simulink model "gm_flyback_dt_vnl"  (R2021b)
settings: Solver=FixedStepDiscrete  StartTime=0.0  StopTime=100e-3  RelTol=1e-3
undefined symbols (not defined in the file or in its folder): DiscIntNeverNeededParam
libraries: simulink x5
Description:
  | Symmetric FIR Filter
  | This example shows how to use HDL Coder(TM) to check, generate,
  | and verify HDL for a fixed-point symmetric FIR filter.
settings Model: Creator=The MathWorks, Inc.  LastModifiedBy=Marco Milanesi
settings SolverCC: AlgebraicLoopSolver=TrustRegion  AutoInsertRateTranBlk=on
settings DataIOCC: LimitDataPoints=on  SaveFormat=Array  SaveOutput=off  SignalLogging=off  SaveTime=off  ReturnWorkspaceOutputs=off  SignalLoggingName=logsOut
settings OptimizationCC: BlockReduction=off  BooleanDataType=off  ConditionallyExecuteInputs=off  DefaultParameterBehavior=Inlined  InheritOutputTypeSmallerThanSingle=on  InlineInvariantSignals=on  ExpressionDepthLimit=2147483647  InitFltsAndDblsToZero=on  LifeSpan=inf  BufferReusableBoundary=off
settings DebuggingCC: AlgebraicLoopMsg=error  SaveWithParameterizedLinksMsg=none  UnderspecifiedInitializationDetection=Classic  MergeDetectMultiDrivingBlocksExec=none  CheckExecutionContextPreStartOutputMsg=on  SignalResolutionControl=TryResolveAllWithWarning  InheritedTsInSrcMsg=none  MultiTaskDSMMsg=warning  MultiTaskCondExecSysMsg=none  SingleTaskRateTransMsg=error  IntegerOverflowMsg=none  ParameterPrecisionLossMsg=none  FcnCallInpInsideContextMsg=warning  BusObjectLabelMismatch=none  StateNameClashWarn=warning  SFUnexpectedBacktrackingDiag=warning  SFNoUnconditionalDefaultTransitionDiag=warning  SFExecutionAtInitializationDiag=none  SFMachineParentedDataDiag=warning  IntegerSaturationMsg=none  ArithmeticOperatorsInVariantConditions=warning
settings HardwareCC: ProdBitPerPointer=32  ProdBitPerSizeT=32  ProdBitPerPtrDiffT=32  ProdLargestAtomicFloat=None  ProdIntDivRoundTo=Undefined  ProdEndianess=Unspecified  ProdWordSize=32  ProdHWDeviceType=ASIC/FPGA  TargetUnknown=on  ProdEqTarget=off
settings ModelReferenceCC: PropagateSignalLabelsOutOfModel=off
settings SFSimCC: SimUseLocalCustomCode=off  CustomCodeUndefinedFunction=UseInterfaceOnly
settings RTWCC: RTWUseLocalCustomCode=off
settings CodeAppCC: StateflowObjectComments=on
settings GRTTargetCC: TargetFcnLib=ansi_tfl_tmw.mat  TargetLangStandard=C89/C90 (ANSI)  CombineOutputUpdateFcns=off  GRTInterface=on
settings ConfigComp: CovMetricSettings=dw  CovSaveCumulativeToWorkspaceVar=on  CovSaveSingleToWorkspaceVar=on  CovExternalEMLEnable=off

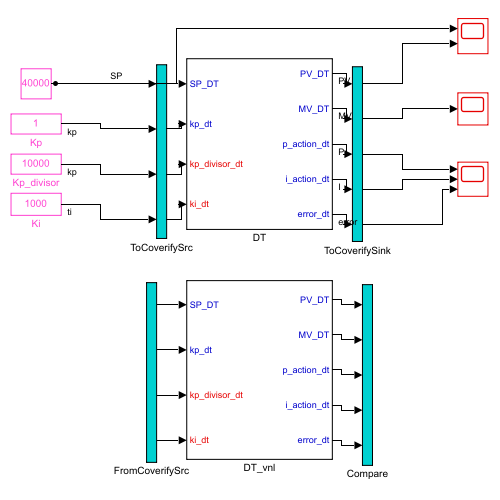
[thumbnail: Simulink's stored preview of the top-level diagram]
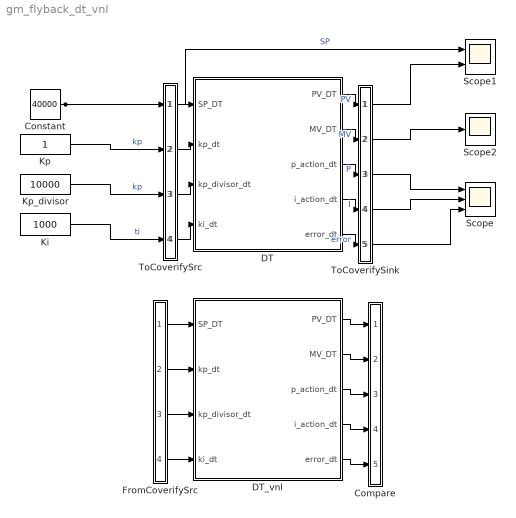
== system gm_flyback_dt_vnl ==
  Compare : Subsystem
      mask Display: disp('')
  Constant : Constant  Value=40000  OutDataTypeStr=fixdt(1,64,32)
  DT : Subsystem
  DT_vnl : Subsystem
  FromCoverifySrc : Subsystem
      mask Display: disp('')
  Ki : Constant  Value=1000  OutDataTypeStr=fixdt(1,64,32)
  Kp : Constant  OutDataTypeStr=fixdt(1,64,32)
  Kp_divisor : Constant  Value=10000  OutDataTypeStr=fixdt(1,64,32)
  Scope : Scope  NumInputPorts=3
  Scope1 : Scope  NumInputPorts=2
  Scope2 : Scope
  ToCoverifySink : Subsystem
      mask Display: disp('')
  ToCoverifySrc : Subsystem
      mask Display: disp('')
  wires:
  Constant/1 -> Scope1/1, ToCoverifySrc/1(in1)  "SP"
  ToCoverifySrc/1(out1) -> DT/1(SP_DT)
  ToCoverifySrc/2(out2) -> DT/2(kp_dt)
  ToCoverifySrc/3(out3) -> DT/3(kp_divisor_dt)
  ToCoverifySrc/4(out4) -> DT/4(ki_dt)
  DT/1(PV_DT) -> ToCoverifySink/1(in1)  "PV"
  DT/2(MV_DT) -> ToCoverifySink/2(in2)  "MV"
  DT/3(p_action_dt) -> ToCoverifySink/3(in3)  "P"
  DT/4(i_action_dt) -> ToCoverifySink/4(in4)  "I"
  DT/5(error_dt) -> ToCoverifySink/5(in5)  "error"
  Kp/1 -> ToCoverifySrc/2(in2)  "kp"
  Kp_divisor/1 -> ToCoverifySrc/3(in3)  "kp"
  Ki/1 -> ToCoverifySrc/4(in4)  "ti"
  ToCoverifySink/1(out1) -> Scope1/2
  ToCoverifySink/2(out2) -> Scope2/1
  ToCoverifySink/3(out3) -> Scope/1
  ToCoverifySink/4(out4) -> Scope/2
  ToCoverifySink/5(out5) -> Scope/3
  FromCoverifySrc/1(out1) -> DT_vnl/1(SP_DT)
  FromCoverifySrc/2(out2) -> DT_vnl/2(kp_dt)
  FromCoverifySrc/3(out3) -> DT_vnl/3(kp_divisor_dt)
  FromCoverifySrc/4(out4) -> DT_vnl/4(ki_dt)
  DT_vnl/1(PV_DT) -> Compare/1(in1)
  DT_vnl/2(MV_DT) -> Compare/2(in2)
  DT_vnl/3(p_action_dt) -> Compare/3(in3)
  DT_vnl/4(i_action_dt) -> Compare/4(in4)
  DT_vnl/5(error_dt) -> Compare/5(in5)

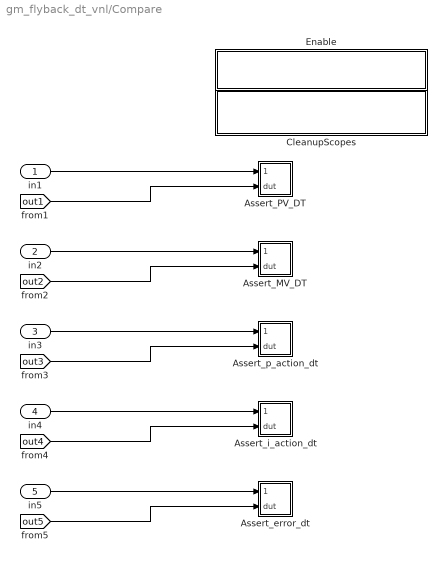
== system gm_flyback_dt_vnl/Compare ==
  in1 : Inport
  in2 : Inport  Port=2
  in3 : Inport  Port=3
  in4 : Inport  Port=4
  in5 : Inport  Port=5
  Assert_MV_DT : Subsystem
  Assert_PV_DT : Subsystem
  Assert_error_dt : Subsystem
  Assert_i_action_dt : Subsystem
  Assert_p_action_dt : Subsystem
  CleanupScopes : Subsystem
      settings: OpenFcn=|
      | blkName = gcb; %self block
      | idx = regexp(blkName, '/CleanupScopes$', 'once');
      | blkParent = blkName(1:idx-1);
      | blks=find_system(blkParent, 'LookUnderMasks', 'all','blocktype', 'Scope');
      | for itr = 1:length(blks)
      | 	 hScopeCfg = get_param(blks{itr},'ScopeConfiguration');
      | 	 hScopeCfg.Visible = ~ hScopeCfg.Visible;
      | end
      | drawnow;
      mask Display: fprintf(message('hdlcoder:cosim:vnl_dblclick').getString());
  Enable : Subsystem
      settings: OpenFcn=|
      | blkName = gcb;
      | idx = regexp(blkName, '/Enable$', 'once');
      | blkParent = blkName(1:idx-1);
      | blks=find_system(blkParent, 'LookUnderMasks', 'all','blocktype', 'Assertion');
      | e = get_param(blks{1}, 'Enabled');
      | if strcmp(e, 'on'), f= 'off';, else, f = 'on';, end
      | for ii=1:length(blks), set_param(blks{ii}, 'Enabled', f);, end
      | set_param(gcb, 'MaskDisplay',['fprintf(message(''hdlcoder:cosim:vnl_dblclick_assertions'',','''',upper(e),'''',').getString())']);
      mask Display: fprintf(message('hdlcoder:cosim:vnl_dblclick_assertions','OFF').getString());
  wires:
  in1/1 -> Assert_PV_DT/1(cosim)
  [out1] -> Assert_PV_DT/2(dut)
  in2/1 -> Assert_MV_DT/1(cosim)
  [out2] -> Assert_MV_DT/2(dut)
  in3/1 -> Assert_p_action_dt/1(cosim)
  [out3] -> Assert_p_action_dt/2(dut)
  in4/1 -> Assert_i_action_dt/1(cosim)
  [out4] -> Assert_i_action_dt/2(dut)
  in5/1 -> Assert_error_dt/1(cosim)
  [out5] -> Assert_error_dt/2(dut)

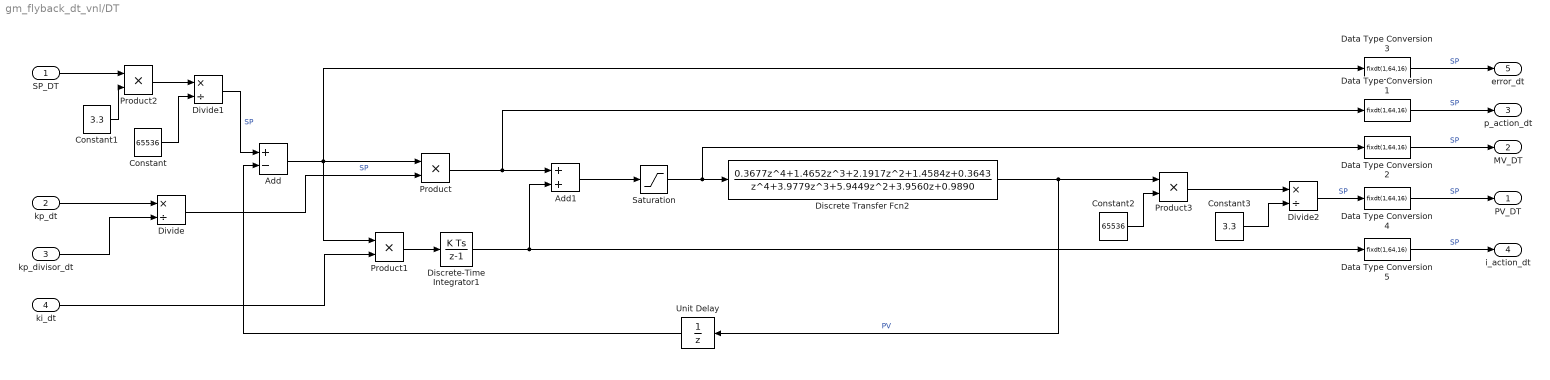
== system gm_flyback_dt_vnl/DT ==
  SP_DT : Inport  OutDataTypeStr=fixdt(1,64,32)  SampleTime=0.00001
  kp_dt : Inport  Port=2  OutDataTypeStr=fixdt(1,64,32)  SampleTime=0.00001
  kp_divisor_dt : Inport  Port=3  OutDataTypeStr=fixdt(1,64,32)  SampleTime=0.00001
  ki_dt : Inport  Port=4  OutDataTypeStr=fixdt(1,64,32)  SampleTime=0.00001
  Add : Sum  Inputs=+-  AccumDataTypeStr=fixdt(1,64,32)  OutDataTypeStr=fixdt(1,64,32)
  Add1 : Sum  AccumDataTypeStr=fixdt(1,64,32)  OutDataTypeStr=fixdt(1,64,32)
  Constant : Constant  Value=65536  OutDataTypeStr=fixdt(1,64,32)
  Constant1 : Constant  Value=3.3  OutDataTypeStr=fixdt(1,64,32)
  Constant2 : Constant  Value=65536  OutDataTypeStr=fixdt(1,64,32)
  Constant3 : Constant  Value=3.3  OutDataTypeStr=fixdt(1,64,32)
  Data Type Conversion{1..5} (5 alike) : DataTypeConversion  OutDataTypeStr=fixdt(1,64,16)
  Discrete Transfer Fcn2 : DiscreteTransferFcn  Numerator=[0.3677 1.4652 2.1917 1.4584 0.3643]  Denominator=[1 3.9779 5.9449 3.9560 0.9890]  SampleTime=0.00001  NumCoefDataTypeStr=fixdt(1,64,32)  DenCoefDataTypeStr=fixdt(1,64,32)  NumProductDataTypeStr=fixdt(1,64,32)  DenProductDataTypeStr=fixdt(1,64,32)  NumAccumDataTypeStr=fixdt(1,64,32)  DenAccumDataTypeStr=fixdt(1,64,32)  OutDataTypeStr=fixdt(1,64,32)
  Discrete-Time Integrator1 : DiscreteIntegrator  SampleTime=0.00001  OutDataTypeStr=fixdt(1,64,32)  ICPrevOutput=DiscIntNeverNeededParam  ICPrevScaledInput=DiscIntNeverNeededParam
  Divide : Product  Inputs=*/  RndMeth=Zero  SaturateOnIntegerOverflow=on  LockScale=on
  Divide1 : Product  Inputs=*/  RndMeth=Zero  SaturateOnIntegerOverflow=on  LockScale=on
  Divide2 : Product  Inputs=*/  RndMeth=Zero  SaturateOnIntegerOverflow=on  LockScale=on
  Product{,1..3} (4 alike) : Product  OutDataTypeStr=fixdt(1,64,32)
  Saturation : Saturate  UpperLimit=255  LowerLimit=0  OutDataTypeStr=fixdt(1,64,32)
  Unit Delay : UnitDelay  SampleTime=0.00001  HasFrameUpgradeWarning=on
  PV_DT : Outport  OutDataTypeStr=fixdt(1,64,16)  SampleTime=0.00001  VectorParamsAs1DForOutWhenUnconnected=off
  MV_DT : Outport  Port=2  OutDataTypeStr=fixdt(1,64,16)  SampleTime=0.00001  VectorParamsAs1DForOutWhenUnconnected=off
  p_action_dt : Outport  Port=3  OutDataTypeStr=fixdt(1,64,16)  SampleTime=0.00001  VectorParamsAs1DForOutWhenUnconnected=off
  i_action_dt : Outport  Port=4  OutDataTypeStr=fixdt(1,64,16)  SampleTime=0.00001  VectorParamsAs1DForOutWhenUnconnected=off
  error_dt : Outport  Port=5  OutDataTypeStr=fixdt(1,64,16)  SampleTime=0.00001  VectorParamsAs1DForOutWhenUnconnected=off
  wires:
  Unit Delay/1 -> Add/2
  Product1/1 -> Discrete-Time Integrator1/1
  Add/1 -> Data Type Conversion3/1, Product/1, Product1/1
  Product/1 -> Data Type Conversion1/1, Add1/1
  Discrete Transfer Fcn2/1 -> Product3/1, Unit Delay/1  "PV"
  Discrete-Time Integrator1/1 -> Data Type Conversion5/1, Add1/2
  Data Type Conversion1/1 -> p_action_dt/1  "SP"
  Data Type Conversion3/1 -> error_dt/1  "SP"
  Data Type Conversion2/1 -> MV_DT/1  "SP"
  Data Type Conversion4/1 -> PV_DT/1  "SP"
  Data Type Conversion5/1 -> i_action_dt/1  "SP"
  ki_dt/1 -> Product1/2
  kp_dt/1 -> Divide/1
  kp_divisor_dt/1 -> Divide/2
  Divide/1 -> Product/2  "SP"
  Add1/1 -> Saturation/1
  Saturation/1 -> Discrete Transfer Fcn2/1, Data Type Conversion2/1
  SP_DT/1 -> Product2/1
  Product2/1 -> Divide1/1
  Divide1/1 -> Add/1  "SP"
  Constant/1 -> Divide1/2
  Constant1/1 -> Product2/2
  Product3/1 -> Divide2/1
  Constant2/1 -> Product3/2
  Constant3/1 -> Divide2/2
  Divide2/1 -> Data Type Conversion4/1  "SP"

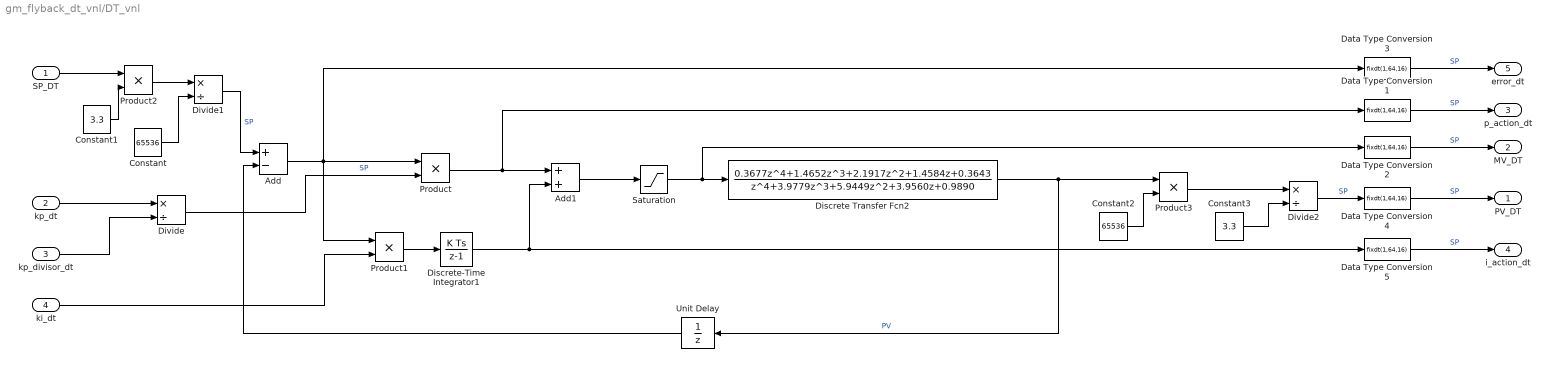
== system gm_flyback_dt_vnl/DT_vnl ==
  SP_DT : Inport  OutDataTypeStr=fixdt(1,64,32)  SampleTime=0.00001
  kp_dt : Inport  Port=2  OutDataTypeStr=fixdt(1,64,32)  SampleTime=0.00001
  kp_divisor_dt : Inport  Port=3  OutDataTypeStr=fixdt(1,64,32)  SampleTime=0.00001
  ki_dt : Inport  Port=4  OutDataTypeStr=fixdt(1,64,32)  SampleTime=0.00001
  Add : Sum  Inputs=+-  AccumDataTypeStr=fixdt(1,64,32)  OutDataTypeStr=fixdt(1,64,32)
  Add1 : Sum  AccumDataTypeStr=fixdt(1,64,32)  OutDataTypeStr=fixdt(1,64,32)
  Constant : Constant  Value=65536  OutDataTypeStr=fixdt(1,64,32)
  Constant1 : Constant  Value=3.3  OutDataTypeStr=fixdt(1,64,32)
  Constant2 : Constant  Value=65536  OutDataTypeStr=fixdt(1,64,32)
  Constant3 : Constant  Value=3.3  OutDataTypeStr=fixdt(1,64,32)
  Data Type Conversion{1..5} (5 alike) : DataTypeConversion  OutDataTypeStr=fixdt(1,64,16)
  Discrete Transfer Fcn2 : DiscreteTransferFcn  Numerator=[0.3677 1.4652 2.1917 1.4584 0.3643]  Denominator=[1 3.9779 5.9449 3.9560 0.9890]  SampleTime=0.00001  NumCoefDataTypeStr=fixdt(1,64,32)  DenCoefDataTypeStr=fixdt(1,64,32)  NumProductDataTypeStr=fixdt(1,64,32)  DenProductDataTypeStr=fixdt(1,64,32)  NumAccumDataTypeStr=fixdt(1,64,32)  DenAccumDataTypeStr=fixdt(1,64,32)  OutDataTypeStr=fixdt(1,64,32)
  Discrete-Time Integrator1 : DiscreteIntegrator  SampleTime=0.00001  OutDataTypeStr=fixdt(1,64,32)  ICPrevOutput=DiscIntNeverNeededParam  ICPrevScaledInput=DiscIntNeverNeededParam
  Divide : Product  Inputs=*/  RndMeth=Zero  SaturateOnIntegerOverflow=on  LockScale=on
  Divide1 : Product  Inputs=*/  RndMeth=Zero  SaturateOnIntegerOverflow=on  LockScale=on
  Divide2 : Product  Inputs=*/  RndMeth=Zero  SaturateOnIntegerOverflow=on  LockScale=on
  Product{,1..3} (4 alike) : Product  OutDataTypeStr=fixdt(1,64,32)
  Saturation : Saturate  UpperLimit=255  LowerLimit=0  OutDataTypeStr=fixdt(1,64,32)
  Unit Delay : UnitDelay  SampleTime=0.00001  HasFrameUpgradeWarning=on
  PV_DT : Outport  OutDataTypeStr=fixdt(1,64,16)  SampleTime=0.00001  VectorParamsAs1DForOutWhenUnconnected=off
  MV_DT : Outport  Port=2  OutDataTypeStr=fixdt(1,64,16)  SampleTime=0.00001  VectorParamsAs1DForOutWhenUnconnected=off
  p_action_dt : Outport  Port=3  OutDataTypeStr=fixdt(1,64,16)  SampleTime=0.00001  VectorParamsAs1DForOutWhenUnconnected=off
  i_action_dt : Outport  Port=4  OutDataTypeStr=fixdt(1,64,16)  SampleTime=0.00001  VectorParamsAs1DForOutWhenUnconnected=off
  error_dt : Outport  Port=5  OutDataTypeStr=fixdt(1,64,16)  SampleTime=0.00001  VectorParamsAs1DForOutWhenUnconnected=off
  wires:
  Divide2/1 -> Data Type Conversion4/1  "SP"
  Constant3/1 -> Divide2/2
  Constant2/1 -> Product3/2
  Product3/1 -> Divide2/1
  Constant1/1 -> Product2/2
  Constant/1 -> Divide1/2
  Divide1/1 -> Add/1  "SP"
  Product2/1 -> Divide1/1
  SP_DT/1 -> Product2/1
  Saturation/1 -> Data Type Conversion2/1, Discrete Transfer Fcn2/1
  Add1/1 -> Saturation/1
  Divide/1 -> Product/2  "SP"
  kp_divisor_dt/1 -> Divide/2
  kp_dt/1 -> Divide/1
  ki_dt/1 -> Product1/2
  Data Type Conversion5/1 -> i_action_dt/1  "SP"
  Data Type Conversion4/1 -> PV_DT/1  "SP"
  Data Type Conversion2/1 -> MV_DT/1  "SP"
  Data Type Conversion3/1 -> error_dt/1  "SP"
  Data Type Conversion1/1 -> p_action_dt/1  "SP"
  Discrete-Time Integrator1/1 -> Add1/2, Data Type Conversion5/1
  Discrete Transfer Fcn2/1 -> Unit Delay/1, Product3/1  "PV"
  Product/1 -> Add1/1, Data Type Conversion1/1
  Add/1 -> Product1/1, Product/1, Data Type Conversion3/1
  Product1/1 -> Discrete-Time Integrator1/1
  Unit Delay/1 -> Add/2

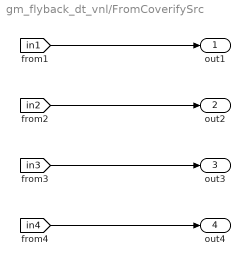
== system gm_flyback_dt_vnl/FromCoverifySrc ==
  out1 : Outport
  out2 : Outport  Port=2
  out3 : Outport  Port=3
  out4 : Outport  Port=4
  wires:
  [in1] -> out1/1
  [in2] -> out2/1
  [in3] -> out3/1
  [in4] -> out4/1

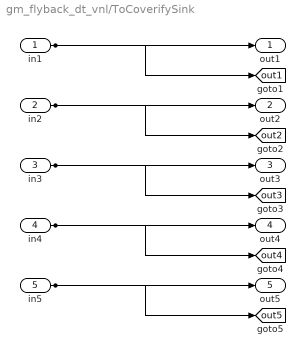
== system gm_flyback_dt_vnl/ToCoverifySink ==
  in1 : Inport
  in2 : Inport  Port=2
  in3 : Inport  Port=3
  in4 : Inport  Port=4
  in5 : Inport  Port=5
  out1 : Outport
  out2 : Outport  Port=2
  out3 : Outport  Port=3
  out4 : Outport  Port=4
  out5 : Outport  Port=5
  tag scope: out1=global, out2=global, out3=global, out4=global, out5=global
  wires:
  in1/1 -> out1/1, [out1]
  in2/1 -> out2/1, [out2]
  in3/1 -> out3/1, [out3]
  in4/1 -> out4/1, [out4]
  in5/1 -> out5/1, [out5]

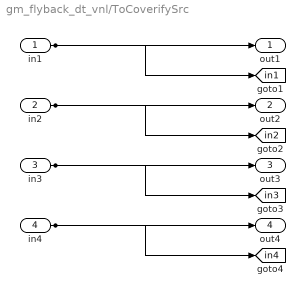
== system gm_flyback_dt_vnl/ToCoverifySrc ==
  in1 : Inport
  in2 : Inport  Port=2
  in3 : Inport  Port=3
  in4 : Inport  Port=4
  out1 : Outport
  out2 : Outport  Port=2
  out3 : Outport  Port=3
  out4 : Outport  Port=4
  tag scope: in1=global, in2=global, in3=global, in4=global
  wires:
  in1/1 -> out1/1, [in1]
  in2/1 -> out2/1, [in2]
  in3/1 -> out3/1, [in3]
  in4/1 -> out4/1, [in4]

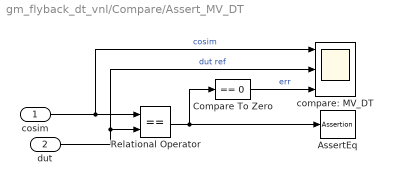
== system gm_flyback_dt_vnl/Compare/Assert_MV_DT ==
  cosim : Inport
  dut : Inport  Port=2
  AssertEq : Assertion  StopWhenAssertionFail=off
  Compare To Zero : simulink/Logic and Bit Operations/Compare To Zero  relop===  OutDataTypeStr=boolean
  Relational Operator : RelationalOperator  Operator===  OutDataTypeStr=boolean  RndMeth=Nearest
  compare: MV_DT : Scope  NumInputPorts=3
  wires:
  Compare To Zero/1 -> compare: MV_DT/3  "err"
  Relational Operator/1 -> Compare To Zero/1, AssertEq/1
  cosim/1 -> compare: MV_DT/1, Relational Operator/1  "cosim"
  dut/1 -> compare: MV_DT/2, Relational Operator/2  "dut ref"

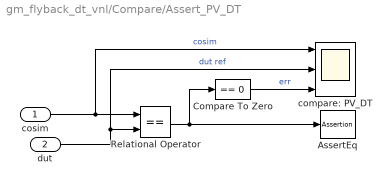
== system gm_flyback_dt_vnl/Compare/Assert_PV_DT ==
  cosim : Inport
  dut : Inport  Port=2
  AssertEq : Assertion  StopWhenAssertionFail=off
  Compare To Zero : simulink/Logic and Bit Operations/Compare To Zero  relop===  OutDataTypeStr=boolean
  Relational Operator : RelationalOperator  Operator===  OutDataTypeStr=boolean  RndMeth=Nearest
  compare: PV_DT : Scope  NumInputPorts=3
  wires:
  Compare To Zero/1 -> compare: PV_DT/3  "err"
  Relational Operator/1 -> Compare To Zero/1, AssertEq/1
  cosim/1 -> compare: PV_DT/1, Relational Operator/1  "cosim"
  dut/1 -> compare: PV_DT/2, Relational Operator/2  "dut ref"

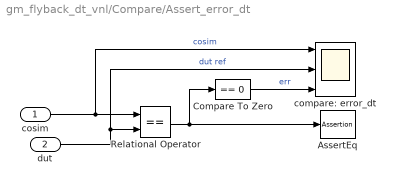
== system gm_flyback_dt_vnl/Compare/Assert_error_dt ==
  cosim : Inport
  dut : Inport  Port=2
  AssertEq : Assertion  StopWhenAssertionFail=off
  Compare To Zero : simulink/Logic and Bit Operations/Compare To Zero  relop===  OutDataTypeStr=boolean
  Relational Operator : RelationalOperator  Operator===  OutDataTypeStr=boolean  RndMeth=Nearest
  compare: error_dt : Scope  NumInputPorts=3
  wires:
  Compare To Zero/1 -> compare: error_dt/3  "err"
  Relational Operator/1 -> Compare To Zero/1, AssertEq/1
  cosim/1 -> compare: error_dt/1, Relational Operator/1  "cosim"
  dut/1 -> compare: error_dt/2, Relational Operator/2  "dut ref"

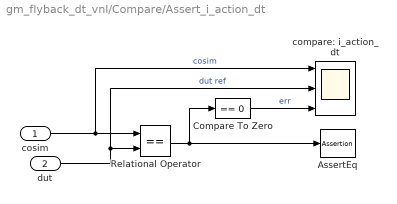
== system gm_flyback_dt_vnl/Compare/Assert_i_action_dt ==
  cosim : Inport
  dut : Inport  Port=2
  AssertEq : Assertion  StopWhenAssertionFail=off
  Compare To Zero : simulink/Logic and Bit Operations/Compare To Zero  relop===  OutDataTypeStr=boolean
  Relational Operator : RelationalOperator  Operator===  OutDataTypeStr=boolean  RndMeth=Nearest
  compare: i_action_dt : Scope  NumInputPorts=3
  wires:
  Compare To Zero/1 -> compare: i_action_dt/3  "err"
  Relational Operator/1 -> Compare To Zero/1, AssertEq/1
  cosim/1 -> compare: i_action_dt/1, Relational Operator/1  "cosim"
  dut/1 -> compare: i_action_dt/2, Relational Operator/2  "dut ref"

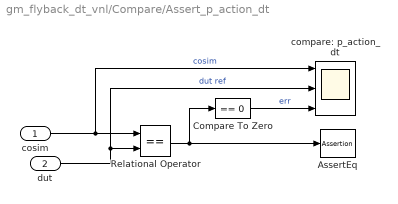
== system gm_flyback_dt_vnl/Compare/Assert_p_action_dt ==
  cosim : Inport
  dut : Inport  Port=2
  AssertEq : Assertion  StopWhenAssertionFail=off
  Compare To Zero : simulink/Logic and Bit Operations/Compare To Zero  relop===  OutDataTypeStr=boolean
  Relational Operator : RelationalOperator  Operator===  OutDataTypeStr=boolean  RndMeth=Nearest
  compare: p_action_dt : Scope  NumInputPorts=3
  wires:
  Compare To Zero/1 -> compare: p_action_dt/3  "err"
  Relational Operator/1 -> Compare To Zero/1, AssertEq/1
  cosim/1 -> compare: p_action_dt/1, Relational Operator/1  "cosim"
  dut/1 -> compare: p_action_dt/2, Relational Operator/2  "dut ref"

== system gm_flyback_dt_vnl/Compare/CleanupScopes ==

== system gm_flyback_dt_vnl/Compare/Enable ==
